simulink model "soc_pmsm_dualcpu_foc"  (R2023b)
settings: Solver=VariableStepAuto  StartTime=0.0  StopTime=.6  RelTol=1e-3  EnableMultiTasking=on
InitFcn:
  | soc_mcb_pmsm_foc_sensorless_f28379d_data;
model workspace (MAT data in the model file):
  mwTaskManagerKernelLatency = 0
values from neighbouring files (symbols this model uses):
  inverter = mcb_SetInverterParameters('BoostXL-DRV8305')    [soc_mcb_pmsm_foc_sensorless_f28379d_data.m]
  pmsm = mcb_SetPMSMMotorParameters('custom')    [soc_mcb_pmsm_foc_sensorless_f28379d_data.m]
  PU_System = mcb_SetPUSystem(pmsm,inverter)    [soc_mcb_pmsm_foc_sensorless_f28379d_data.m]
  PWM_frequency = 20e3    (= 20000)    [soc_mcb_pmsm_foc_sensorless_f28379d_data.m]
  Ts_motor = T_pwm/2    (= 2.5e-05)    [soc_mcb_pmsm_foc_sensorless_f28379d_data.m]
undefined symbols (not defined in the file or in its folder): D1, D2, Down, m, n, P, Up
libraries: fl_lib x50, nesl_utility x15, ee_lib x11, peripheralslib x5, procinterlib x2, proctasklib x2, mcbplantlib x1, mcbpositiondecoderlib x1, autolibpmsmexterior x1
(part 1 of 2)
settings Model: ExtModeTrigDuration=8  Creator=The MathWorks, Inc.  LastModifiedBy=The MathWorks, Inc.
settings SolverCC: AlgebraicLoopSolver=TrustRegion  PositivePriorityOrder=on  MaxZcPerStep=1
settings DataIOCC: SaveOutput=off  DSMLogging=off
settings OptimizationCC: DefaultUnderspecifiedDataType=single  EnhancedBackFolding=on  PassReuseOutputArgsAs=Individual arguments  MaxStackSize=1024  OptimizeBlockOrder=speed  DifferentSizesBufferReuse=on  OptimizationCustomize=off  DenormalBehavior=FlushToZero  EfficientTunableParamExpr=on
settings DebuggingCC: ParameterPrecisionLossMsg=none  ParameterTunabilityLossMsg=error  UnconnectedInputMsg=warning  UnconnectedOutputMsg=warning  UnconnectedLineMsg=warning
settings HardwareCC: ProdBitPerChar=16  ProdBitPerInt=16  ProdBitPerPointer=32  ProdBitPerSizeT=32  ProdBitPerPtrDiffT=32  ProdLargestAtomicInteger=Integer  ProdLargestAtomicFloat=None  ProdWordSize=16  ProdLongLongMode=on  ProdHWDeviceType=Texas Instruments->C2000  HardwareBoardFeatureSet=SoCBlockset
settings ModelReferenceCC: EnableRefExpFcnMdlSchedulingChecks=on
settings SFSimCC: MATLABDynamicMemAlloc=off
settings RTWCC: Description=Embedded Coder  SystemTargetFile=ert.tlc  HardwareBoard=TI Delfino F28379D LaunchPad  TLCOptions="-aInlineSetEventsForThisBaseRateFcn=TLC_FALSE -aSuppressMultiTaskScheduler=TLC_FALSE   -aRateBasedStepFcn=1"  TemplateMakefile=ert_default_tmf  Toolchain=Texas Instruments Code Composer Studio (C2000)  DLArmComputeVersion=19.05
settings CodeAppCC: ForceParamTrailComments=on  IgnoreCustomStorageClasses=off  OperatorAnnotations=on  SimulinkDataObjDesc=on  SFDataObjDesc=on  InsertBlockDesc=on
settings ERTTargetCC: CodeReplacementLibrary=TI C28x  ExtModeStaticAllocSize=10000

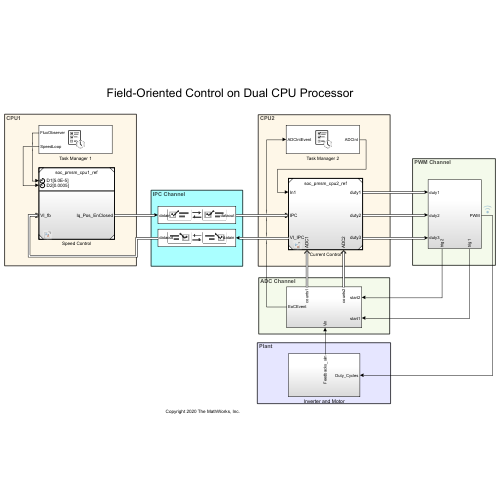
[thumbnail: Simulink's stored preview of the top-level diagram]
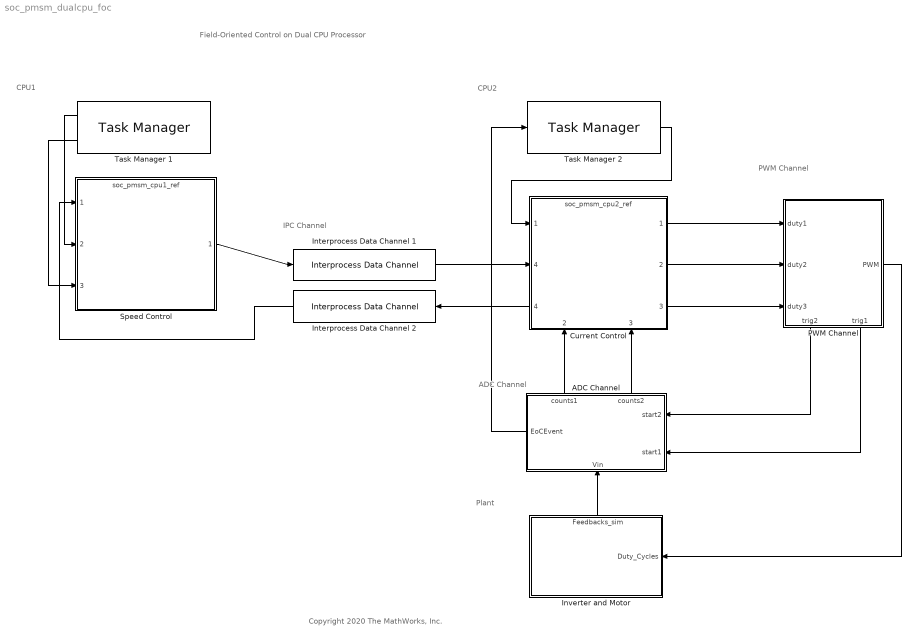
== system soc_pmsm_dualcpu_foc ==
  note: Field-Oriented Control on Dual CPU Processor
  note: CPU1
  note: PWM Channel
  note: IPC Channel
  note: CPU2
  note: Plant
  note: ADC Channel
  note: Copyright 2020 The MathWorks, Inc.
  ADC Channel : Subsystem
      settings: PortSchema="{\"entries\":[{\"content\":{\"sides\":[{\"content\":{\"connectorIds\":[\"In1\"]},\"type\":\"ConnectorPlacement.EquallySpacedRectSide\",\"uuid\":\"667350c5-41cd-4cba-abc8-8d5d0ac94845\"},{\"content\":{\"connectorIds\":[\"Out1\",\"Out2\"],\"side\":\"RIGHT\"},\"type\":\"ConnectorPlacement.EquallySpacedRectSide\",\"uuid\":\"5a172c81-9350-4ccc-b7f4-df82d7eca1de\"},{\"content\":{\"connectorIds\":[\"Out3\"],\"side\":\"TOP\"},\"type\":\"ConnectorPlacement.EquallySpacedRectSide\",\"uuid\":\"3830ed3a-e235-4bdf-8511-f25666678fd6\"},{\"content\":{\"connectorIds\":[\"In2\",\"In3\"],\"side\":\"BOTTOM\"},\"type\":\"ConnectorPlacement.EquallySpacedRectSide\",\"uuid\":\"15f45d0c-0c23-40c1-aa04-14d3d7fcf92d\"},{\"content\":{\"connectorIds\":[],\"side\":\"HIDDEN\"},\"type\":\"ConnectorPlacement.EquallySpacedRectSide\",\"uuid\":\"ee7e5474-69fd-4152-9972-ad3b7eda0b9e\"}]},\"type\":\"ConnectorPlacement.EquallySpacedConnector\",\"uuid\":\"8c4cca9e-82dc-4501-bb7e-3f52a3bf47b4\"}],\"packageUris\":[\"http://schema.mathworks.com/mf0/Connector/R2020b\"],\"version\":\"1.0\"}"
  Current Control : ModelReference  InputPortMessageModes=n,m,m,m  OutputPortMessageModes=m,m,m,m  ModelNameDialog=soc_pmsm_cpu2_ref.slx  SimulationMode=Normal  CachedPortDiscreteRates=[0.2]  ModelReferenceVersion=8.0
      settings: PortSchema="{\"entries\":[{\"content\":{\"sides\":[{\"content\":{\"connectorIds\":[\"In1\",\"In4\",\"Out4\"]},\"type\":\"ConnectorPlacement.EquallySpacedRectSide\",\"uuid\":\"9fd2c24c-ae51-46e5-a431-71bc240ed721\"},{\"content\":{\"connectorIds\":[\"Out1\",\"Out2\",\"Out3\"],\"side\":\"RIGHT\"},\"type\":\"ConnectorPlacement.EquallySpacedRectSide\",\"uuid\":\"f0a0e173-5aee-453c-b1bd-b370cde086ab\"},{\"content\":{\"connectorIds\":[],\"side\":\"TOP\"},\"type\":\"ConnectorPlacement.EquallySpacedRectSide\",\"uuid\":\"79c8d290-c938-4b10-a214-67592e778693\"},{\"content\":{\"connectorIds\":[\"In2\",\"In3\"],\"side\":\"BOTTOM\"},\"type\":\"ConnectorPlacement.EquallySpacedRectSide\",\"uuid\":\"f9ab5770-0d25-45e9-9b4a-55a67569c63a\"},{\"content\":{\"connectorIds\":[],\"side\":\"HIDDEN\"},\"type\":\"ConnectorPlacement.EquallySpacedRectSide\",\"uuid\":\"b923878a-78df-441a-99e2-7ad72d4d69ab\"}]},\"type\":\"ConnectorPlacement.EquallySpacedConnector\",\"uuid\":\"a5006b0b-636b-4340-a85c-125b87b251fa\"}],\"packageUris\":[\"http://schema.mathworks.com/mf0/Connector/R2020b\"],\"version\":\"1.0\"}"
  Interprocess Data Channel 1 : procinterlib/Interprocess Data Channel  NumBuffers=1  PropagationDelay=0  ShowEventPort=off  ShowNumUsedBuffers=off  ShowBufferOverwritten=off
  Interprocess Data Channel 2 : procinterlib/Interprocess Data Channel  NumBuffers=1  PropagationDelay=0  ShowEventPort=off  ShowNumUsedBuffers=off  ShowBufferOverwritten=off
  Inverter and Motor : Subsystem
      settings: PortSchema="{\"entries\":[{\"content\":{\"sides\":[{\"content\":{\"connectorIds\":[\"In1\"]},\"type\":\"ConnectorPlacement.EquallySpacedRectSide\",\"uuid\":\"958970e8-f51f-4be6-a255-39048d8abc04\"},{\"content\":{\"connectorIds\":[],\"side\":\"RIGHT\"},\"type\":\"ConnectorPlacement.EquallySpacedRectSide\",\"uuid\":\"a7d67471-63de-4fa9-8929-71ac779bb3a0\"},{\"content\":{\"connectorIds\":[\"Out1\"],\"side\":\"TOP\"},\"type\":\"ConnectorPlacement.EquallySpacedRectSide\",\"uuid\":\"f6853a86-6c38-405e-966d-f0bd0978db63\"},{\"content\":{\"connectorIds\":[],\"side\":\"HIDDEN\"},\"type\":\"ConnectorPlacement.EquallySpacedRectSide\",\"uuid\":\"0017b626-46a9-47f1-bc71-1e5fb05a995f\"}]},\"type\":\"ConnectorPlacement.EquallySpacedConnector\",\"uuid\":\"d320a7cc-19d6-4ac2-b759-0c9b58a9d13f\"}],\"packageUris\":[\"http://schema.mathworks.com/mf0/Connector/R2020b\"],\"version\":\"1.0\"}"
  PWM Channel : Subsystem
      settings: PortSchema="{\"entries\":[{\"content\":{\"sides\":[{\"content\":{\"connectorIds\":[\"In1\",\"In2\",\"In3\"]},\"type\":\"ConnectorPlacement.EquallySpacedRectSide\",\"uuid\":\"93269d63-2f51-4397-8262-c0fba5a35fbc\"},{\"content\":{\"connectorIds\":[\"Out1\"],\"side\":\"RIGHT\"},\"type\":\"ConnectorPlacement.EquallySpacedRectSide\",\"uuid\":\"01a9fb74-5fff-4873-a961-955e91d37141\"},{\"content\":{\"connectorIds\":[],\"side\":\"TOP\"},\"type\":\"ConnectorPlacement.EquallySpacedRectSide\",\"uuid\":\"96774146-0690-4e4a-a90b-a04dbe81855e\"},{\"content\":{\"connectorIds\":[\"Out2\",\"Out3\"],\"side\":\"BOTTOM\"},\"type\":\"ConnectorPlacement.EquallySpacedRectSide\",\"uuid\":\"cc316efe-bea7-4750-8d36-9fcd57c23279\"},{\"content\":{\"connectorIds\":[],\"side\":\"HIDDEN\"},\"type\":\"ConnectorPlacement.EquallySpacedRectSide\",\"uuid\":\"75c797b2-ef98-4bb8-8ad0-83cc5de0a8e5\"}]},\"type\":\"ConnectorPlacement.EquallySpacedConnector\",\"uuid\":\"6875c10b-95f0-453b-a724-f824d2af4c4b\"}],\"packageUris\":[\"http://schema.mathworks.com/mf0/Connector/R2020b\"],\"version\":\"1.0\"}"
  Speed Control : ModelReference  InputPortMessageModes=m,n,n  OutputPortMessageModes=m  ModelNameDialog=soc_pmsm_cpu1_ref.slx  SimulationMode=Normal  ScheduleRates=on  CachedPortDiscreteRates=[5.0E-5;0.0005]  ModelEventPortInfo=P:D1[5.0E-5][0][0],P:D2[0.0005][0][0]  ModelReferenceVersion=8.0
  Task Manager 1 : proctasklib/Task Manager  AllTaskData="[{\"taskName\":\"FluxObserver\",\"taskType\":\"Timer-driven\",\"taskEvent\":\"SpeedEvent\",\"taskPeriod\":\"Ts\",\"taskPriority\":\"50\",\"coreSelection\":\"Specified core\",\"coreNum\":\"0\",\"dropOverranTasks\":false,\"playbackRecorded\":false,\"diagnosticsFile\":\"\",\"taskDurationSource\":\"Dialog\",\"taskDuration\":1E-6,\"taskDurationDeviation\":0,\"logExecutionData\":true,\"logDroppedTasks\":false,\"version\":\"2.6\",\"taskDurationData\":{\"percent\":\"100\",\"mean\":\"1e-06\",\"dev\":\"0\",\"min\":\"1e-06\",\"max\":\"1e-06\"},\"taskEventSource\":\"Internal\",\"taskEventSourceAssignmentType\":\"AutoAssigned\",\"taskEventSourceType\":\"Unspecified\",\"taskEventGroup\":\"Unspecified\",\"taskEventInterrupt\":\"Unspecified\",\"taskEventOrder\":1,\"taskDisablePremption\":false,\"taskClearInterruptFlagsAtEndOfEvent\":false},{\"taskName\":\"SpeedLoop\",\"taskType\":\"Timer-driven\",\"taskEvent\":\"newTask1Event\",\"taskPeriod\":\"Ts_speed\",\"taskPriority\":\"50\",\"coreSelection\":\"Specified core\",\"coreNum\":\"0\",\"dropOverranTasks\":false,\"playbackRecorded\":false,\"diagnosticsFile\":\"\",\"taskDurationSource\":\"Dialog\",\"taskDuration\":1E-6,\"taskDurationDeviation\":0,\"logExecutionData\":true,\"logDroppedTasks\":false,\"version\":\"2.6\",\"taskDurationData\":{\"percent\":\"100\",\"mean\":\"1e-06\",\"dev\":\"0\",\"min\":\"1e-06\",\"max\":\"1e-06\"},\"taskEventSource\":\"Internal\",\"taskEventSourceAssignmentType\":\"AutoAssigned\",\"taskEventSourceType\":\"Unspecified\",\"taskEventGroup\":\"Unspecified\",\"taskEventInterrupt\":\"Unspecified\",\"taskEventOrder\":1,\"taskDisablePremption\":false,\"taskClearInterruptFlagsAtEndOfEvent\":false}]"  EnableTaskSimulation=off  StreamToSDI=on  WriteToFile=off  OverwriteFile=off  SupportEventPorts=on  UseScheduleEditor=off  CustomizationInfo=''
  Task Manager 2 : proctasklib/Task Manager  AllTaskData="{\"taskName\":\"ADCInt\",\"taskType\":\"Event-driven\",\"taskEvent\":\"ADCIntEvent\",\"taskPeriod\":\"0.1\",\"taskPriority\":\"50\",\"coreSelection\":\"Specified core\",\"coreNum\":\"0\",\"dropOverranTasks\":false,\"playbackRecorded\":false,\"diagnosticsFile\":\"\",\"taskDurationSource\":\"Dialog\",\"taskDuration\":1E-6,\"taskDurationDeviation\":0,\"logExecutionData\":true,\"logDroppedTasks\":false,\"version\":\"2.6\",\"taskDurationData\":{\"percent\":\"100\",\"mean\":\"1e-06\",\"dev\":\"0\",\"min\":\"1e-06\",\"max\":\"1e-06\"},\"taskEventSource\":\"EOC event\",\"taskEventSourceAssignmentType\":\"ManuallyAssigned\",\"taskEventSourceType\":\"Unspecified\",\"taskEventGroup\":\"ADC - Analog to Digital Converter\",\"taskEventInterrupt\":\"ADCB1_INT\",\"taskEventOrder\":1,\"taskDisablePremption\":false,\"taskClearInterruptFlagsAtEndOfEvent\":false}"  EnableTaskSimulation=off  StreamToSDI=on  WriteToFile=off  OverwriteFile=off  SupportEventPorts=on  UseScheduleEditor=off  CustomizationInfo=''
  wires:
  Speed Control/1 -> Interprocess Data Channel 1/1
  Interprocess Data Channel 2/1 -> Speed Control/1
  PWM Channel/1(PWM) -> Inverter and Motor/1(Duty_Cycles)
  ADC Channel/3(EoCEvent) -> Task Manager 2/1
  Task Manager 2/1 -> Current Control/1
  PWM Channel/2(trig2) -> ADC Channel/3(start2)
  PWM Channel/3(trig1) -> ADC Channel/2(start1)
  Interprocess Data Channel 1/1 -> Current Control/4
  Inverter and Motor/1(Feedbacks_sim) -> ADC Channel/1(Vin)
  ADC Channel/1(counts1) -> Current Control/2
  ADC Channel/2(counts2) -> Current Control/3
  Current Control/4 -> Interprocess Data Channel 2/1
  Current Control/1 -> PWM Channel/1(duty1)
  Current Control/2 -> PWM Channel/2(duty2)
  Current Control/3 -> PWM Channel/3(duty3)
  Task Manager 1/1 -> Speed Control/2
  Task Manager 1/2 -> Speed Control/3

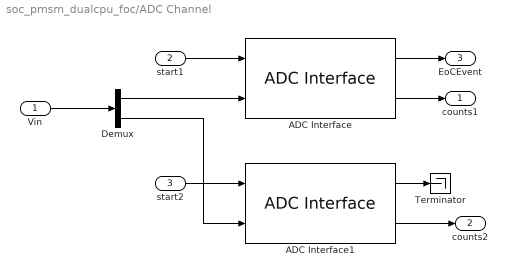
== system soc_pmsm_dualcpu_foc/ADC Channel ==
  Vin : Inport
  start1 : Inport  Port=2
  start2 : Inport  Port=3
  ADC Interface : peripheralslib/ADC Interface  ADCResolution=12  HighVref=3  AcqTime=320e-9  ConvTime=240e-9  TimeConstant=40e-9  SoftTrig=off  SampleTime=1e-3  NumCh=1  ConvType=Sequential  EnInterrupt=on  IntCondition=Acquisition + Conversion time  EnWatchdog=off  LowThreshold=.1  HighThreshold=2.9  IntLatency=0
  ADC Interface1 : peripheralslib/ADC Interface  ADCResolution=12  HighVref=3  AcqTime=320e-9  ConvTime=240e-9  TimeConstant=40e-9  SoftTrig=off  SampleTime=1e-3  NumCh=1  ConvType=Sequential  EnInterrupt=on  IntCondition=Acquisition + Conversion time  EnWatchdog=off  LowThreshold=.1  HighThreshold=2.9  IntLatency=0
  Demux : Demux  Outputs=2
  Terminator : Terminator
  counts1 : Outport
  counts2 : Outport  Port=2
  EoCEvent : Outport  Port=3
  wires:
  start1/1 -> ADC Interface/1
  start2/1 -> ADC Interface1/1
  Demux/2 -> ADC Interface1/2
  Vin/1 -> Demux/1
  Demux/1 -> ADC Interface/2
  ADC Interface1/2 -> counts2/1
  ADC Interface1/1 -> Terminator/1
  ADC Interface/2 -> counts1/1
  ADC Interface/1 -> EoCEvent/1

== system soc_pmsm_dualcpu_foc/Inverter and Motor ==
  Duty_Cycles : Inport
  Average or Switching : Subsystem  Variant=on  VariantControlMode=label  LabelModeActiveChoice=AverageInverter
  Feedbacks_sim : Outport  VectorParamsAs1DForOutWhenUnconnected=off
  wires:
  Average or Switching/1(Feedbacks_sim) -> Feedbacks_sim/1
  Duty_Cycles/1 -> Average or Switching/1(Duty_Cycles)

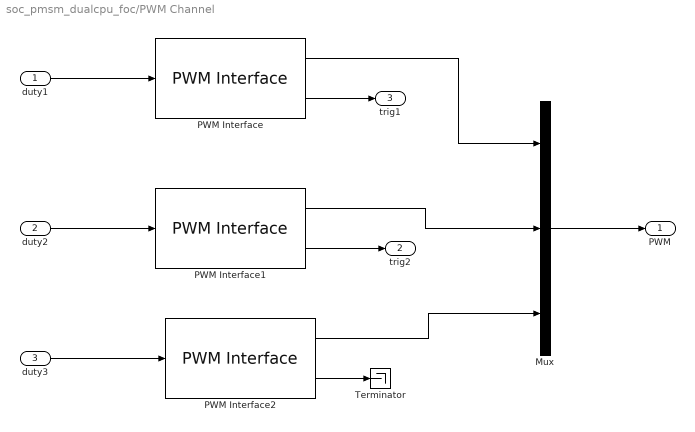
== system soc_pmsm_dualcpu_foc/PWM Channel ==
  duty1 : Inport
  duty2 : Inport  Port=2
  duty3 : Inport  Port=3
  Mux : Mux  Inputs=3
  PWM Interface : peripheralslib/PWM Interface  Period=1/PWM_frequency  OutSigMode=Average  CounterMode=Up-Down  GenCompPWM=off  DeadTimeTopPWM=100e-9  DeadTimeBottomPWM=100e-9  EventCondition2=End of PWM period  DataType=single  PWMAtStartPeriod=High  PWMAtMidPeriod=NoChange  PWMAtCMP1=Low  PWMAtCMP1UpCnt=Low  PWMAtCMP1DwnCnt=High  PWMAtCMP2=NoChange  PWMAtCMP2UpCnt=NoChange  PWMAtCMP2DwnCnt=NoChange  OutCountDir=off  PhaseOffset=0  EventType=ADC start  EventCondition1=Mid of PWM period  NumADCSOCToWait=1st event  NumADCSOCReplica=1  InterruptCond=End of PWM period  IntLatency=0  NumInterruptToWait=1st event
      settings: SamplingMode=End of PWM period
  PWM Interface1 : peripheralslib/PWM Interface  Period=1/PWM_frequency  OutSigMode=Average  CounterMode=Up-Down  GenCompPWM=off  DeadTimeTopPWM=100e-9  DeadTimeBottomPWM=100e-9  EventCondition2=End of PWM period  DataType=single  PWMAtStartPeriod=High  PWMAtMidPeriod=NoChange  PWMAtCMP1=Low  PWMAtCMP1UpCnt=Low  PWMAtCMP1DwnCnt=High  PWMAtCMP2=NoChange  PWMAtCMP2UpCnt=NoChange  PWMAtCMP2DwnCnt=NoChange  OutCountDir=off  PhaseOffset=0  EventType=ADC start  EventCondition1=Mid of PWM period  NumADCSOCToWait=1st event  NumADCSOCReplica=1  InterruptCond=End of PWM period  IntLatency=0  NumInterruptToWait=1st event
      settings: SamplingMode=End of PWM period
  PWM Interface2 : peripheralslib/PWM Interface  Period=1/PWM_frequency  OutSigMode=Average  CounterMode=Up-Down  GenCompPWM=off  DeadTimeTopPWM=100e-9  DeadTimeBottomPWM=100e-9  EventCondition2=End of PWM period  DataType=single  PWMAtStartPeriod=High  PWMAtMidPeriod=NoChange  PWMAtCMP1=Low  PWMAtCMP1UpCnt=Low  PWMAtCMP1DwnCnt=High  PWMAtCMP2=NoChange  PWMAtCMP2UpCnt=NoChange  PWMAtCMP2DwnCnt=NoChange  OutCountDir=off  PhaseOffset=0  EventType=ADC start  EventCondition1=Mid of PWM period  NumADCSOCToWait=1st event  NumADCSOCReplica=1  InterruptCond=End of PWM period  IntLatency=0  NumInterruptToWait=1st event
      settings: SamplingMode=End of PWM period
  Terminator : Terminator
  PWM : Outport
  trig2 : Outport  Port=2
  trig1 : Outport  Port=3
  wires:
  PWM Interface/2 -> trig1/1
  PWM Interface1/2 -> trig2/1
  PWM Interface2/2 -> Terminator/1
  Mux/1 -> PWM/1
  PWM Interface/1 -> Mux/1
  PWM Interface1/1 -> Mux/2
  PWM Interface2/1 -> Mux/3
  duty1/1 -> PWM Interface/1
  duty2/1 -> PWM Interface1/1
  duty3/1 -> PWM Interface2/1

== system soc_pmsm_dualcpu_foc/Inverter and Motor/Average or Switching ==
  note: 1) Add Subsystem or Model blocks as valid variant choices.
      | 2) You cannot connect blocks at this level. At simulation, connectivity is automatically
      | determined, based on the active variant and port name matching.
  Duty_Cycles : Inport
  Average : Subsystem  VariantControl=AverageInverter
  Switching : Subsystem  VariantControl=SwitchingInverter
  Feedbacks_sim : Outport  VectorParamsAs1DForOutWhenUnconnected=off

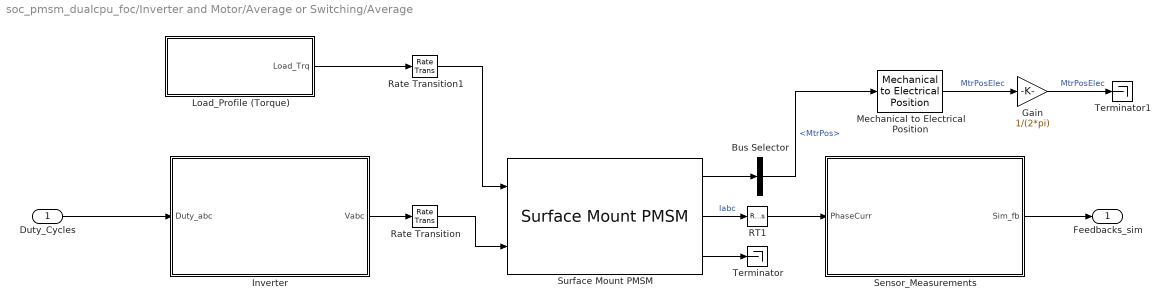
== system soc_pmsm_dualcpu_foc/Inverter and Motor/Average or Switching/Average ==
  Duty_Cycles : Inport
  Bus Selector : BusSelector  OutputSignals=MtrPos
  Gain : Gain  Gain=1/(2*pi)  OutDataTypeStr=Inherit: Same as input
  Inverter : Subsystem
  Load_Profile (Torque) : Subsystem
  Mechanical to Electrical Position : mcbpositiondecoderlib/Mechanical to Electrical Position  PolePairsInputType=Specify via dialog  NrPP=pmsm.p  selectedRange=Radians  MechOfstInputType=Specify via dialog  mechOffsetIn=0  maxAngleIn=2*pi  InputDataType=single  VariantSelect=floating-point
  RT1 : RateTransition  Deterministic=off  OutPortSampleTime=Ts_simulink
  Rate Transition : RateTransition  Deterministic=off  OutPortSampleTime=Ts_motor
  Rate Transition1 : RateTransition  Deterministic=off  OutPortSampleTime=Ts_motor
  Sensor_Measurements : Subsystem
  Surface Mount PMSM : autolibpmsmexterior/Surface Mount PMSM  port_config=Torque  sim_type=Discrete  Ts=Ts_motor  FilePath=surfacepmsm_motordata.m  P=pmsm.p  Rs=pmsm.Rs + inverter.R_board  Ldq_=pmsm.Ld  KConstText=Permanent flux linkage constant (lambda_pm):  lambda_pm=pmsm.FluxPM  Ke=159.9771  Kt=1.323  mechanical=[pmsm.J, pmsm.B, 0]  idq0=[0 0]  theta_init=0  omega_init=0  KConst=pmsm.FluxPM  lambda_pm_calc=pmsm.FluxPM  RefBlkName='autolibpmsmexterior/Surface Mount PMSM'  aMode=5  Ldq="[0.0002      0.0002]"
  Terminator : Terminator
  Terminator1 : Terminator
  Feedbacks_sim : Outport  VectorParamsAs1DForOutWhenUnconnected=off
  wires:
  Rate Transition/1 -> Surface Mount PMSM/2
  Gain/1 -> Terminator1/1  "MtrPosElec"
  Inverter/1(Vabc) -> Rate Transition/1
  Load_Profile (Torque)/1(Load_Trq) -> Rate Transition1/1
  RT1/1 -> Sensor_Measurements/1(PhaseCurr)
  Surface Mount PMSM/1 -> Bus Selector/1
  Bus Selector/1 -> Mechanical to Electrical Position/1  "<MtrPos>"
  Duty_Cycles/1 -> Inverter/1(Duty_abc)
  Surface Mount PMSM/2 -> RT1/1  "Iabc"
  Mechanical to Electrical Position/1 -> Gain/1  "MtrPosElec"
  Sensor_Measurements/1(Sim_fb) -> Feedbacks_sim/1
  Rate Transition1/1 -> Surface Mount PMSM/1
  Surface Mount PMSM/3 -> Terminator/1

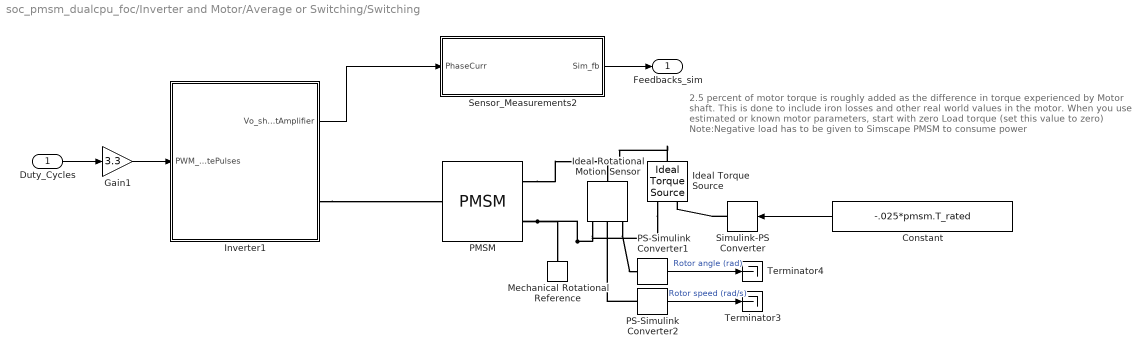
== system soc_pmsm_dualcpu_foc/Inverter and Motor/Average or Switching/Switching ==
  note: 2.5 percent of motor torque is roughly added as the difference in torque experienced by Motor shaft. This is done to include iron losses and other real world values in the motor.
      |
      | When you use estimated or known motor parameters, start with zero Load torque (set this value to zero)
      |
      | Note:Negative load has to be given to  Simscape PMSM to consume power
  Duty_Cycles : Inport
  Constant : Constant  Value=-.025*pmsm.T_rated  OutDataTypeStr=double
  Gain1 : Gain  Gain=3.3
  Ideal Rotational Motion Sensor : fl_lib/Mechanical/Mechanical Sensors/Ideal Rotational Motion Sensor  reference=foundation.enum.MeasurementReference.difference  acceleration_port=false  velocity_port=true  position_port=true  wrap_angle=simscape.enum.onoff.off  offset=0 deg
  Ideal Torque Source : fl_lib/Mechanical/Mechanical Sources/Ideal Torque Source
  Inverter1 : Subsystem
  Mechanical Rotational Reference : fl_lib/Mechanical/Rotational Elements/Mechanical Rotational Reference
  PMSM : ee_lib/Electromechanical/Permanent Magnet/PMSM  port_option=ee.enum.threePhasePort.composite  winding_type=ee.enum.statorconnection.wye  machine_param=ee.enum.pmsm.parameterization.constant  nPolePairs=pmsm.p  pmflux_param=ee.enum.pmflux.fluxlinkage  pm_flux_linkage=pmsm.FluxPM Wb  torque_constant=0.18 N*m/A  back_emf_constant=0.18 V/(rad/s)  stator_param=ee.enum.statorparam.LdLqL0  Ld=pmsm.Ld H  Lq=pmsm.Ld H  idVec=[-200, 0, 200] A  iqVec=[-200, 0, 200] A  LdMatrix=0.0002 * ones(3, 3) H  LqMatrix=0.0002 * ones(3, 3) H  PmMatrix=0.1 * ones(3, 3) Wb  ktMatrix=0.18 * ones(3, 3) N*m/A  keMatrix=0.18 * ones(3, 3) V/(rad/s)  L0=0 H  Ls=0.0002 H  Lm=-0.00002 H  Ms=0.00002 H  Rs=pmsm.Rs + inverter.R_board Ohm  zero_sequence=ee.enum.park.zerosequence.exclude  axes_param=ee.enum.rotorangle.daxis  loss_param=ee.enum.ironloss.none  losses_oc=[0, 0, 0] W  losses_sc=[0, 0, 0] W  f_losses=60 Hz  Isc_losses=95 A  J=pmsm.J kg*m^2  lam=pmsm.B N*m/(rad/s)  i_d_specify=off  i_d_priority=None  i_d=0 A  i_d_nominal_specify=off  i_d_nominal_unit=A  i_d_nominal_value=1  i_q_specify=off  i_q_priority=None  i_q=0 A  i_q_nominal_specify=off  i_q_nominal_unit=A  i_q_nominal_value=1  torque_specify=off  torque_priority=None  torque=0 N*m  torque_nominal_specify=off  torque_nominal_unit=N*m  torque_nominal_value=1  angular_velocity_specify=off  angular_velocity_priority=High  angular_velocity=0 rpm  angular_velocity_nominal_specify=off  angular_velocity_nominal_unit=rpm  angular_velocity_nominal_value=1  angular_position_specify=off  angular_position_priority=High  angular_position=0 deg  angular_position_nominal_specify=off  angular_position_nominal_unit=deg  angular_position_nominal_value=1  alpha=3.93e-3 1/K  alpha_flux=-0.001 1/K  Tmeas=298.15 K  stator_thermal_mass=100 J/K  rotor_thermal_mass=200 J/K  Rm_percent_rotor=90  Rd_percent_rotor=30  temperatureA_specify=off  temperatureA_priority=High  temperatureA=25 degC  temperatureA_nominal_specify=off  temperatureA_nominal_unit=degC  temperatureA_nominal_value=1  temperatureB_specify=off  temperatureB_priority=High  temperatureB=25 degC  temperatureB_nominal_specify=off  temperatureB_nominal_unit=degC  temperatureB_nominal_value=1  temperatureC_specify=off  temperatureC_priority=High  temperatureC=25 degC  temperatureC_nominal_specify=off  temperatureC_nominal_unit=degC  temperatureC_nominal_value=1  temperatureR_specify=off  temperatureR_priority=High  temperatureR=25 degC  temperatureR_nominal_specify=off  temperatureR_nominal_unit=degC  temperatureR_nominal_value=1
      settings: InternalSimscapePortConfiguration="{\"Bottom\":[],\"Left\":[{\"id\":\"N\",\"label\":\"~\",\"type\":\"foundation.electrical.three_phase\"}],\"Right\":[{\"id\":\"R\",\"label\":\"R\",\"type\":\"foundation.mechanical.rotational.rotational\"},{\"id\":\"C\",\"label\":\"C\",\"type\":\"foundation.mechanical.rotational.rotational\"}],\"Top\":[]}"
  PS-Simulink Converter1 : nesl_utility/PS-Simulink Converter  PhysicalDomain=network_engine_domain  SubClassName=ps_output  LeftPortType=input  RightPortType=output  PseudoPeriodic=off  Frequencies=[]  VectorFormat=1-D array  Unit=rad  AffineConversion=off
  PS-Simulink Converter2 : nesl_utility/PS-Simulink Converter  PhysicalDomain=network_engine_domain  SubClassName=ps_output  LeftPortType=input  RightPortType=output  PseudoPeriodic=off  Frequencies=[]  VectorFormat=1-D array  Unit=rad/s  AffineConversion=off
  Sensor_Measurements2 : Subsystem
  Simulink-PS Converter : nesl_utility/Simulink-PS Converter  PhysicalDomain=network_engine_domain  SubClassName=ps_input  LeftPortType=input  RightPortType=output  PseudoPeriodic=off  Frequencies=[]  NoiseDistribution=none  NoiseParameters=[]  Unit=1  AffineConversion=off  FilteringAndDerivatives=provide  SimscapeFilterOrder=1  InputFilterTimeConstant=0.001  UdotUserProvided=0
  Terminator3 : Terminator
  Terminator4 : Terminator
  Feedbacks_sim : Outport  VectorParamsAs1DForOutWhenUnconnected=off
  wires:
  Inverter1/1(Vo_shuntAmplifier) -> Sensor_Measurements2/1(PhaseCurr)
  Gain1/1 -> Inverter1/1(PWM_GatePulses)
  PS-Simulink Converter2/1 -> Terminator3/1  "Rotor speed (rad/s)"
  PS-Simulink Converter1/1 -> Terminator4/1  "Rotor angle (rad)"
  Duty_Cycles/1 -> Gain1/1
  Sensor_Measurements2/1(Sim_fb) -> Feedbacks_sim/1
  Constant/1 -> Simulink-PS Converter/1
  connections:
  PMSM/RConn1 -- Ideal Rotational Motion Sensor/LConn1 -- Ideal Torque Source/LConn1
  PMSM/RConn2 -- Mechanical Rotational Reference/LConn1 -- Ideal Rotational Motion Sensor/RConn1 -- Ideal Torque Source/RConn2
  PS-Simulink Converter2/LConn1 -- Ideal Rotational Motion Sensor/RConn2
  Inverter1/RConn1 -- PMSM/LConn1
  Ideal Rotational Motion Sensor/RConn3 -- PS-Simulink Converter1/LConn1
  Simulink-PS Converter/RConn1 -- Ideal Torque Source/RConn1

== system soc_pmsm_dualcpu_foc/Inverter and Motor/Average or Switching/Average/Inverter ==
  Duty_abc : Inport
  Average-Value Inverter : mcbplantlib/Average-Value Inverter
  Constant2 : Constant  Value=inverter.V_dc  OutDataTypeStr=single  SampleTime=-1
  Data Type Conversion1 : DataTypeConversion  OutDataTypeStr=single  RndMeth=Simplest  SaturateOnIntegerOverflow=off
  Rate Transition3 : RateTransition  Deterministic=off  OutPortSampleTime=Ts_inverter
  Vabc : Outport  VectorParamsAs1DForOutWhenUnconnected=off
  wires:
  Data Type Conversion1/1 -> Rate Transition3/1
  Duty_abc/1 -> Data Type Conversion1/1
  Rate Transition3/1 -> Average-Value Inverter/1
  Constant2/1 -> Average-Value Inverter/2
  Average-Value Inverter/1 -> Vabc/1

== system soc_pmsm_dualcpu_foc/Inverter and Motor/Average or Switching/Average/Load_Profile (Torque) ==
  note: 2.5 percent of motor torque is roughly added as the difference in torque experienced by Motor shaft. This is done to include iron losses and other real world values in the motor.
      |
      | When you use estimated or known motor parameters, start with zero Load torque (set this value to zero)
  Constant : Constant  Value=.025*pmsm.T_rated  OutDataTypeStr=single
  Load_Trq : Outport  VectorParamsAs1DForOutWhenUnconnected=off
  wires:
  Constant/1 -> Load_Trq/1

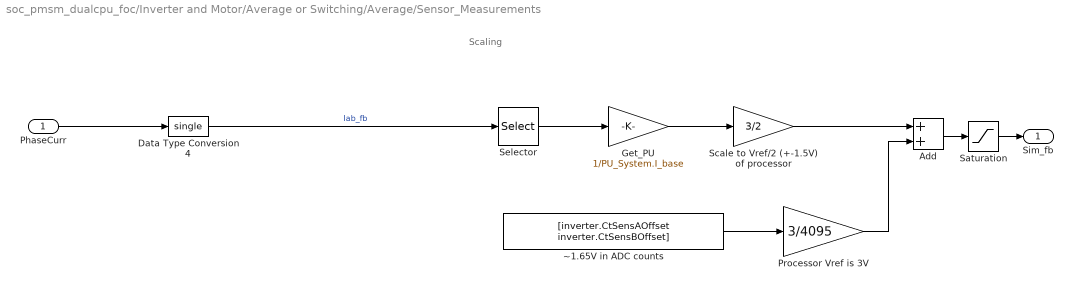
== system soc_pmsm_dualcpu_foc/Inverter and Motor/Average or Switching/Average/Sensor_Measurements ==
  note: Scaling
  PhaseCurr : Inport
  Add : Sum
  Data Type Conversion4 : DataTypeConversion  OutDataTypeStr=single  RndMeth=Simplest  SaturateOnIntegerOverflow=off
  Get_PU : Gain  Gain=1/PU_System.I_base  RndMeth=Simplest
  Processor Vref is 3V : Gain  Gain=3/4095  OutDataTypeStr=single
  Saturation : Saturate  UpperLimit=3.3  LowerLimit=0
  Scale to Vref/2 (+-1.5V) of processor : Gain  Gain=3/2  RndMeth=Simplest  OutDataTypeStr=Inherit: Same as input
  Selector : Selector  InputPortWidth=3  IndexOptions=Index vector (dialog)  Indices=[1 2]  OutputSizes=1
  ~1.65V in ADC counts : Constant  Value=[inverter.CtSensAOffset inverter.CtSensBOffset]  OutDataTypeStr=uint16  SampleTime=-1
  Sim_fb : Outport  VectorParamsAs1DForOutWhenUnconnected=off
  wires:
  Add/1 -> Saturation/1
  ~1.65V in ADC counts/1 -> Processor Vref is 3V/1
  Data Type Conversion4/1 -> Selector/1  "Iab_fb"
  Selector/1 -> Get_PU/1
  PhaseCurr/1 -> Data Type Conversion4/1
  Get_PU/1 -> Scale to Vref/2 (+-1.5V) of processor/1
  Processor Vref is 3V/1 -> Add/2
  Saturation/1 -> Sim_fb/1
  Scale to Vref/2 (+-1.5V) of processor/1 -> Add/1

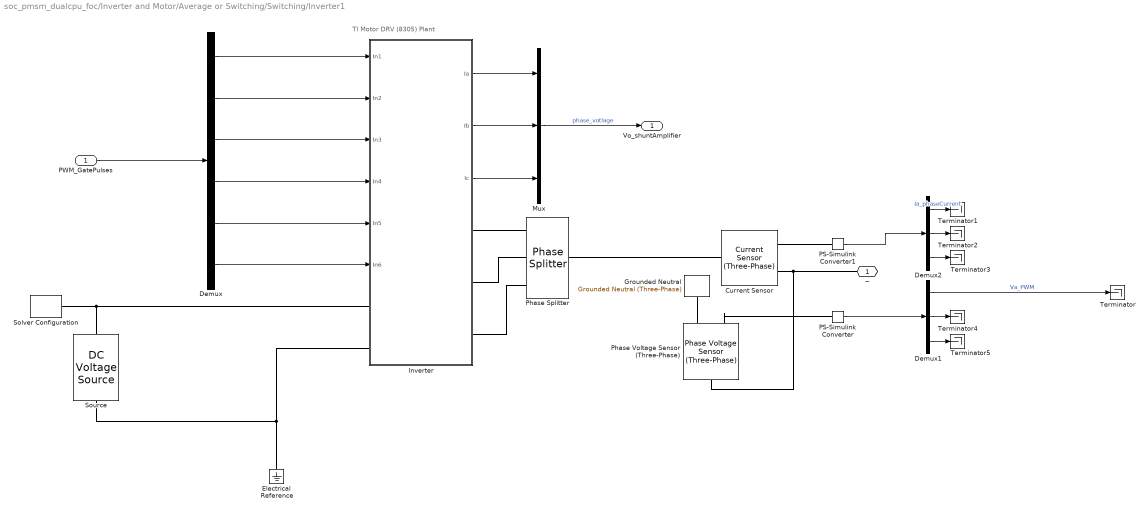
== system soc_pmsm_dualcpu_foc/Inverter and Motor/Average or Switching/Switching/Inverter1 ==
  note: TI Motor DRV (8305) Plant
  PWM_GatePulses : Inport
  Current Sensor : ee_lib/Sensors & Transducers/Current Sensor (Three-Phase)
  Demux : Demux  Outputs=6
  Demux1 : Demux  Outputs=3
  Demux2 : Demux  Outputs=3
  Electrical Reference : fl_lib/Electrical/Electrical Elements/Electrical Reference
  Grounded Neutral : ee_lib/Connectors & References/Grounded Neutral (Three-Phase)
  Inverter : Subsystem
  Mux : Mux  Inputs=3
  PS-Simulink Converter : nesl_utility/PS-Simulink Converter  PhysicalDomain=network_engine_domain  SubClassName=ps_output  LeftPortType=input  RightPortType=output  PseudoPeriodic=off  Frequencies=[]  VectorFormat=1-D array  Unit=1  AffineConversion=off
  PS-Simulink Converter1 : nesl_utility/PS-Simulink Converter  PhysicalDomain=network_engine_domain  SubClassName=ps_output  LeftPortType=input  RightPortType=output  PseudoPeriodic=off  Frequencies=[]  VectorFormat=1-D array  Unit=1  AffineConversion=off
  Phase Splitter : ee_lib/Connectors & References/Phase Splitter
  Phase Voltage Sensor (Three-Phase) : ee_lib/Sensors & Transducers/Phase Voltage Sensor (Three-Phase)
  Solver Configuration : nesl_utility/Solver Configuration  PhysicalDomain=network_engine_domain  SubClassName=solver  LeftPortType=input  RightPortType=generic  Tones=[]  Harmonics=[]  SimulateNoise=off  Profile=off  UseLocalSampling=off  EnableSwitchedLinearOptims=on  FrequencyDomain=off  UseCCode=off  RelTol=0.001  AbsTol=1e-06  MinStep=1e-09  ToWorkspace=off  RevertToSquareIcSolve=off  NumHomotopyIterations=100  PhasorMode=off  PhasorModeNumHarmonics=1  ConsistencySolver=NEWTON_FTOL  IndexReductionMethod=DerivativeReplacement  DoDC=off  ResidualTolerance=1e-09  ConsistencyTolSource=GLOBAL  ConsistencyAbsTol=0.001  ConsistencyRelTol=0.001  ConsistencyTolFactor=0.001  UseLocalSolver=off  LocalSolverChoice=NE_BACKWARD_EULER_ADVANCER  ResolveIndetEquations=on  FunctionEvalNumThread=1  LocalSolverSampleTime=.5e-6  DoFixedCost=off  MaxNonlinIter=3  MaxModeIter=2  ComputeImpulses=off  ImpulseIterations=1  LinearAlgebra=auto  LinearAlgebraNumThread=0  EquationFormulation=NE_TIME_EF  DelaysMemoryBudget=1024  AutomaticFiltering=on  FilteringTimeConstant=0.001  PartitionStorageMethod=AS_NEEDED  PartitionMemoryBudget=1024  PartitionMethod=ROBUST  MultibodyUseLocalSolver=off  MultibodyLocalSolverChoice=ODE1  MultibodyLocalSolverSampleTime=0.001
  Source : fl_lib/Electrical/Electrical Sources/DC Voltage Source  v0=inverter.V_dc V
  Terminator{,1..5} (6 alike) : Terminator
  ~ : PMIOPort  Side=Right
  Vo_shuntAmplifier : Outport  VectorParamsAs1DForOutWhenUnconnected=off
  wires:
  PWM_GatePulses/1 -> Demux/1
  Mux/1 -> Vo_shuntAmplifier/1  "phase_votlage"
  PS-Simulink Converter/1 -> Demux1/1
  PS-Simulink Converter1/1 -> Demux2/1
  Demux2/1 -> Terminator1/1  "Ia_phaseCurrent"
  Inverter/3(Ic) -> Mux/3
  Inverter/1(Ia) -> Mux/1
  Inverter/2(Ib) -> Mux/2
  Demux2/2 -> Terminator2/1
  Demux2/3 -> Terminator3/1
  Demux1/2 -> Terminator4/1
  Demux1/3 -> Terminator5/1
  Demux1/1 -> Terminator/1  "Va_PWM"
  Demux/1 -> Inverter/1(In1)
  Demux/2 -> Inverter/2(In2)
  Demux/3 -> Inverter/3(In3)
  Demux/4 -> Inverter/4(In4)
  Demux/5 -> Inverter/5(In5)
  Demux/6 -> Inverter/6(In6)
  connections:
  Current Sensor/LConn1 -- Phase Splitter/LConn1
  Grounded Neutral/LConn1 -- Phase Voltage Sensor (Three-Phase)/RConn2
  Phase Voltage Sensor (Three-Phase)/RConn1 -- PS-Simulink Converter/LConn1
  Current Sensor/RConn1 -- PS-Simulink Converter1/LConn1
  Source/LConn1 -- Solver Configuration/RConn1 -- Inverter/LConn1
  Electrical Reference/LConn1 -- Inverter/LConn2 -- Source/RConn1
  ~/RConn1 -- Phase Voltage Sensor (Three-Phase)/LConn1 -- Current Sensor/RConn2
  Inverter/RConn3 -- Phase Splitter/RConn3
  Inverter/RConn2 -- Phase Splitter/RConn2
  Inverter/RConn1 -- Phase Splitter/RConn1

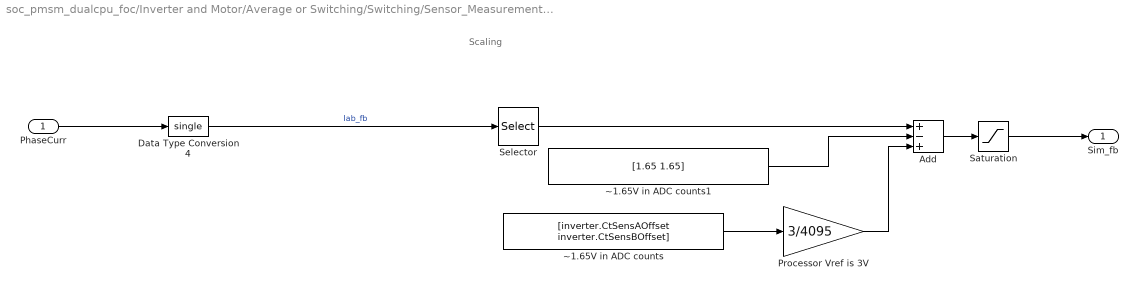
== system soc_pmsm_dualcpu_foc/Inverter and Motor/Average or Switching/Switching/Sensor_Measurements2 ==
  note: Scaling
  PhaseCurr : Inport
  Add : Sum  Inputs=+-+
  Data Type Conversion4 : DataTypeConversion  OutDataTypeStr=single  RndMeth=Simplest  SaturateOnIntegerOverflow=off
  Processor Vref is 3V : Gain  Gain=3/4095  OutDataTypeStr=single
  Saturation : Saturate  UpperLimit=3  LowerLimit=0
  Selector : Selector  InputPortWidth=3  IndexOptions=Index vector (dialog)  Indices=[1 2]  OutputSizes=1
  ~1.65V in ADC counts : Constant  Value=[inverter.CtSensAOffset inverter.CtSensBOffset]  OutDataTypeStr=uint16  SampleTime=-1
  ~1.65V in ADC counts1 : Constant  Value=[1.65 1.65]  OutDataTypeStr=single  SampleTime=-1
  Sim_fb : Outport  VectorParamsAs1DForOutWhenUnconnected=off
  wires:
  Add/1 -> Saturation/1
  ~1.65V in ADC counts/1 -> Processor Vref is 3V/1
  Data Type Conversion4/1 -> Selector/1  "Iab_fb"
  PhaseCurr/1 -> Data Type Conversion4/1
  Saturation/1 -> Sim_fb/1
  Selector/1 -> Add/1
  Processor Vref is 3V/1 -> Add/3
  ~1.65V in ADC counts1/1 -> Add/2

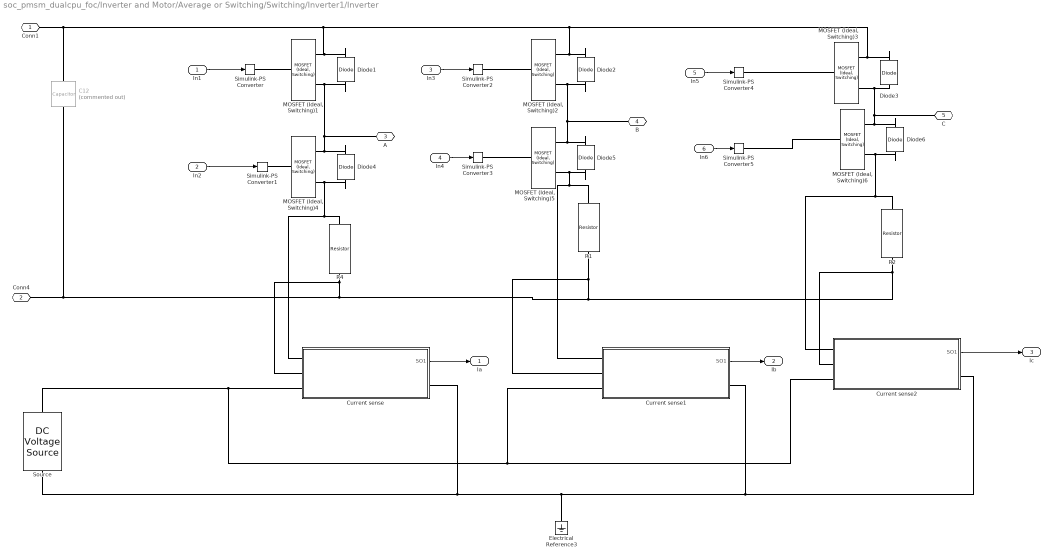
== system soc_pmsm_dualcpu_foc/Inverter and Motor/Average or Switching/Switching/Inverter1/Inverter ==
  In1 : Inport
  In2 : Inport  Port=2
  In3 : Inport  Port=3
  In4 : Inport  Port=4
  In5 : Inport  Port=5
  In6 : Inport  Port=6
  C12 : fl_lib/Electrical/Electrical Elements/Capacitor  Commented=on  c=5000 pF  r=1e-6 Ohm  g=0 1/Ohm  i_specify=off  i_priority=None  i=0 A  i_nominal_specify=off  i_nominal_unit=A  i_nominal_value=1  v_specify=off  v_priority=None  v=0 V  v_nominal_specify=off  v_nominal_unit=V  v_nominal_value=1  vc_specify=off  vc_priority=High  vc=0 V  vc_nominal_specify=off  vc_nominal_unit=V  vc_nominal_value=1
  Current sense : Subsystem
  Current sense1 : Subsystem
  Current sense2 : Subsystem
  Diode{1..6} (6 alike) : fl_lib/Electrical/Electrical Elements/Diode  Vf=.7 V  Ron=1e-6 Ohm  Goff=1e-8 1/Ohm  i_specify=off  i_priority=None  i=0 A  i_nominal_specify=off  i_nominal_unit=A  i_nominal_value=1  v_specify=off  v_priority=None  v=0 V  v_nominal_specify=off  v_nominal_unit=V  v_nominal_value=1
  Electrical Reference3 : fl_lib/Electrical/Electrical Elements/Electrical Reference
  MOSFET (Ideal, Switching){1..6} (6 alike) : ee_lib/Semiconductors & Converters/MOSFET (Ideal, Switching)  port_option=ee.enum.controlport.ps  Rds=2.6e-3 Ohm  Goff=1e-6 1/Ohm  Vth=2 V  diode_param=1  diode_Vf=0.8 V  diode_Ron=0.001 Ohm  diode_Goff=1e-5 1/Ohm  diode_C=50e-9 F  diode_iRM=-235 A  diode_iF=300 A  diode_idot=-50 A/us  diode_trr_param=1  diode_trr_factor=3  diode_trr=15 us  diode_Qrr=1500 s*uA  ids_specify=off  ids_priority=None  ids=0 A  ids_nominal_specify=off  ids_nominal_unit=A  ids_nominal_value=1  vds_specify=off  vds_priority=None  vds=0 V  vds_nominal_specify=off  vds_nominal_unit=V  vds_nominal_value=1  vgs_specify=off  vgs_priority=None  vgs=0 V  vgs_nominal_specify=off  vgs_nominal_unit=V  vgs_nominal_value=1  thermal_loss_option=ee.enum.converters.thermalLossOption.constantvalues  Von_data=[0, 1.8, 3.2, 6, 10, 16; 0, 2, 5.5, 9.5, 15, 25] V  Tj=[298.15, 448.15] K  Iout_data=[0, 20, 40, 60, 80, 100] A  Eon_data=[0, 55.04, 124.57, 235.53, 362.12; 0, 71.25, 161.25, 304.88, 468.75] * 1e-6 J  Eoff_data=[0, 18, 30, 56.1, 76.5; 0, 22.5, 37.5, 70.13, 95.63] * 1e-6 J  Eon_data_3D=[zeros(2, 5, 3)] J  Eoff_data_3D=[zeros(2, 5, 3)] J  Tj_loss=[298.15, 448.15] K  Iout_data_loss=[0, 10, 20, 30, 40] A  tabulateWithVds=false  Vds_loss=[0, 150, 300] V  Eon_scalar=22.86e-3 J  Eoff_scalar=17.14e-3 J  Voff=300 V  Iout_scalar=600 A  useCurrentFromPreviousCycle=false  useVoltageFromPreviousCycle=false  diodeModelType=ee.enum.converters.diodeModelType.pwl  diodeTableType=ee.enum.diode.tableType.IfMat  diode_IfMat=[.07, .12, .19, 1.75, 4.24, 7.32, 11.2; .16, .3, .72, 2.14, 4.02, 6.35, 9.12] A  diode_VfMat=[.9, 1.15, 1.25, 1.5, 1.75, 2.17, 2.6, 2.85; .58, .68, .75, 1.1, 1.38, 1.77, 2.27, 2.7] V  diode_TjVec=[25, 125] degC  diode_VfVec=[.5, .7, .9, 1.3, 1.7, 2.1, 2.5] V  diode_IfVec=[.1, .2, .5, 1, 2, 4, 7, 10] A  diode_Vr=-600 V  diode_Ls=150 nH  diode_Erec=0.03 J  diode_rec_loss_model=ee.enum.diode.reverseRecoveryModel.fixed  diode_ErecVal=0 J  diode_scaleWithIandV=true  diode_ErecMat=zeros(2, 3) J  diode_TjrecVec=[298.15, 398.15] K  diode_IfrecVec=[.1, 1, 10] A  diode_IrecVal=10 A  diode_VrecVal=10 V  diode_tFilter=1 / 1000 / 100 s  thermal_network_parameterization=ee.enum.thermalNetworkTopology.external  Rth=[.03, .2] K/W  Rth_Cauer=[.03, .1, .2] K/W  Rth_Foster=[.03, .2] K/W  thermal_mass_parameterization=ee.enum.thermalNetwork.timeconstant  thermal_mass=[3, 25] J/K  thermal_mass_Cauer=[3, 10, 25] J/K  thermal_mass_Foster=[33, 50] J/K  thermal_time_constant=[.1, 5] s  thermal_time_constant_Cauer=[.1, 1, 5] s  thermal_time_constant_Foster=[1, 10] s  thermal_mass_initial_temperatures=[25, 25] degC  thermal_mass_initial_temperatures_Cauer=[25, 25, 25] degC  junction_thermal_mass=0.1 J/K  Tvec_initial_Foster=[25, 25, 25, 25] degC  no_thermal_network=0  junction_temperature_specify=off  junction_temperature_priority=None  junction_temperature=25 degC  junction_temperature_nominal_specify=off  junction_temperature_nominal_unit=degC  junction_temperature_nominal_value=1  Qj_specify=off  Qj_priority=None  Qj=0 W  Qj_nominal_specify=off  Qj_nominal_unit=W  Qj_nominal_value=1  accumulatedSwitchingLosses_specify=off  accumulatedSwitchingLosses_priority=None  accumulatedSwitchingLosses=0 J
  R1 : fl_lib/Electrical/Electrical Elements/Resistor  R=.007 Ohm  i_specify=off  i_priority=None  i=0 A  i_nominal_specify=off  i_nominal_unit=A  i_nominal_value=1  v_specify=off  v_priority=None  v=0 V  v_nominal_specify=off  v_nominal_unit=V  v_nominal_value=1
  R2 : fl_lib/Electrical/Electrical Elements/Resistor  R=.007 Ohm  i_specify=off  i_priority=None  i=0 A  i_nominal_specify=off  i_nominal_unit=A  i_nominal_value=1  v_specify=off  v_priority=None  v=0 V  v_nominal_specify=off  v_nominal_unit=V  v_nominal_value=1
  R4 : fl_lib/Electrical/Electrical Elements/Resistor  R=.007 Ohm  i_specify=off  i_priority=None  i=0 A  i_nominal_specify=off  i_nominal_unit=A  i_nominal_value=1  v_specify=off  v_priority=None  v=0 V  v_nominal_specify=off  v_nominal_unit=V  v_nominal_value=1
  Simulink-PS Converter{,1..5} (6 alike) : nesl_utility/Simulink-PS Converter  PhysicalDomain=network_engine_domain  SubClassName=ps_input  LeftPortType=input  RightPortType=output  PseudoPeriodic=off  Frequencies=[]  NoiseDistribution=none  NoiseParameters=[]  Unit=1  AffineConversion=off  FilteringAndDerivatives=provide  SimscapeFilterOrder=1  InputFilterTimeConstant=0.001  UdotUserProvided=0
  Source : fl_lib/Electrical/Electrical Sources/DC Voltage Source  v0=3.3 V
  Conn1 : PMIOPort  Side=Left
  Conn4 : PMIOPort  Port=2  Side=Left
  A : PMIOPort  Port=3  Side=Right
  B : PMIOPort  Port=4  Side=Right
  C : PMIOPort  Port=5  Side=Right
  Ia : Outport  VectorParamsAs1DForOutWhenUnconnected=off
  Ib : Outport  Port=2  VectorParamsAs1DForOutWhenUnconnected=off
  Ic : Outport  Port=3  VectorParamsAs1DForOutWhenUnconnected=off
  wires:
  In5/1 -> Simulink-PS Converter4/1
  In4/1 -> Simulink-PS Converter3/1
  In3/1 -> Simulink-PS Converter2/1
  In2/1 -> Simulink-PS Converter1/1
  Current sense1/1(SO1) -> Ib/1
  Current sense/1(SO1) -> Ia/1
  Current sense2/1(SO1) -> Ic/1
  In6/1 -> Simulink-PS Converter5/1
  In1/1 -> Simulink-PS Converter/1
  connections:
  Diode4/LConn1 -- Current sense/LConn1 -- R4/LConn1 -- "MOSFET (Ideal, Switching)4"/RConn2
  Conn4/RConn1 -- R1/RConn1 -- Current sense1/LConn2 -- Current sense2/LConn2 -- R2/RConn1 -- R4/RConn1 -- Current sense/LConn2 -- C12/RConn1
  Diode5/LConn1 -- R1/LConn1 -- Current sense1/LConn1 -- "MOSFET (Ideal, Switching)5"/RConn2
  Diode6/LConn1 -- R2/LConn1 -- Current sense2/LConn1 -- "MOSFET (Ideal, Switching)6"/RConn2
  Current sense1/LConn3 -- Current sense2/LConn3 -- Current sense/LConn3 -- Source/LConn1
  Current sense1/RConn1 -- Current sense2/RConn1 -- Electrical Reference3/LConn1 -- Source/RConn1 -- Current sense/RConn1
  Diode2/RConn1 -- "MOSFET (Ideal, Switching)1"/RConn1 -- Diode1/RConn1 -- C12/LConn1 -- Conn1/RConn1 -- "MOSFET (Ideal, Switching)3"/RConn1 -- Diode3/RConn1 -- "MOSFET (Ideal, Switching)2"/RConn1
  Diode4/RConn1 -- "MOSFET (Ideal, Switching)1"/RConn2 -- Diode1/LConn1 -- A/RConn1 -- "MOSFET (Ideal, Switching)4"/RConn1
  Diode5/RConn1 -- B/RConn1 -- "MOSFET (Ideal, Switching)2"/RConn2 -- Diode2/LConn1 -- "MOSFET (Ideal, Switching)5"/RConn1
  Simulink-PS Converter/RConn1 -- "MOSFET (Ideal, Switching)1"/LConn1
  Simulink-PS Converter1/RConn1 -- "MOSFET (Ideal, Switching)4"/LConn1
  "MOSFET (Ideal, Switching)5"/LConn1 -- Simulink-PS Converter3/RConn1
  Diode6/RConn1 -- C/RConn1 -- Diode3/LConn1 -- "MOSFET (Ideal, Switching)3"/RConn2 -- "MOSFET (Ideal, Switching)6"/RConn1
  Simulink-PS Converter4/RConn1 -- "MOSFET (Ideal, Switching)3"/LConn1
  Simulink-PS Converter5/RConn1 -- "MOSFET (Ideal, Switching)6"/LConn1
  Simulink-PS Converter2/RConn1 -- "MOSFET (Ideal, Switching)2"/LConn1

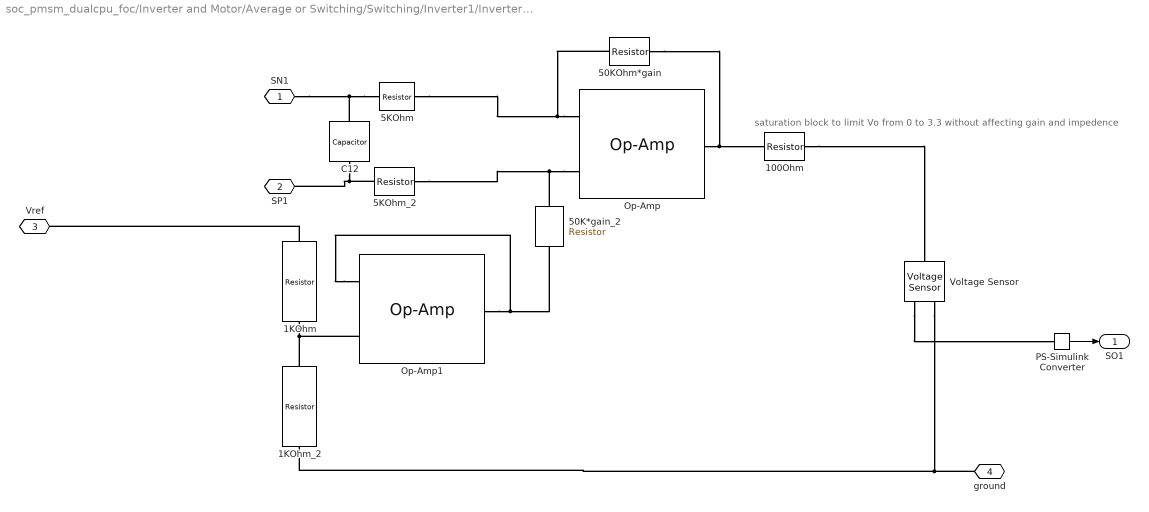
== system soc_pmsm_dualcpu_foc/Inverter and Motor/Average or Switching/Switching/Inverter1/Inverter/Current sense ==
  note: saturation block to limit Vo from 0 to 3.3 without affecting gain and impedence
  100Ohm : fl_lib/Electrical/Electrical Elements/Resistor  R=100 Ohm  i_specify=off  i_priority=None  i=0 A  i_nominal_specify=off  i_nominal_unit=A  i_nominal_value=1  v_specify=off  v_priority=None  v=0 V  v_nominal_specify=off  v_nominal_unit=V  v_nominal_value=1
  1KOhm : fl_lib/Electrical/Electrical Elements/Resistor  R=1 kOhm  i_specify=off  i_priority=None  i=0 A  i_nominal_specify=off  i_nominal_unit=A  i_nominal_value=1  v_specify=off  v_priority=None  v=0 V  v_nominal_specify=off  v_nominal_unit=V  v_nominal_value=1
  1KOhm_2 : fl_lib/Electrical/Electrical Elements/Resistor  R=1 kOhm  i_specify=off  i_priority=None  i=0 A  i_nominal_specify=off  i_nominal_unit=A  i_nominal_value=1  v_specify=off  v_priority=None  v=0 V  v_nominal_specify=off  v_nominal_unit=V  v_nominal_value=1
  50K*gain_2 : fl_lib/Electrical/Electrical Elements/Resistor  R=50*inverter.ADCGain kOhm  i_specify=off  i_priority=None  i=0 A  i_nominal_specify=off  i_nominal_unit=A  i_nominal_value=1  v_specify=off  v_priority=None  v=0 V  v_nominal_specify=off  v_nominal_unit=V  v_nominal_value=1
  50KOhm*gain : fl_lib/Electrical/Electrical Elements/Resistor  R=50*inverter.ADCGain kOhm  i_specify=off  i_priority=None  i=0 A  i_nominal_specify=off  i_nominal_unit=A  i_nominal_value=1  v_specify=off  v_priority=None  v=0 V  v_nominal_specify=off  v_nominal_unit=V  v_nominal_value=1
  5KOhm : fl_lib/Electrical/Electrical Elements/Resistor  R=5 kOhm  i_specify=off  i_priority=None  i=0 A  i_nominal_specify=off  i_nominal_unit=A  i_nominal_value=1  v_specify=off  v_priority=None  v=0 V  v_nominal_specify=off  v_nominal_unit=V  v_nominal_value=1
  5KOhm_2 : fl_lib/Electrical/Electrical Elements/Resistor  R=5 kOhm  i_specify=off  i_priority=None  i=0 A  i_nominal_specify=off  i_nominal_unit=A  i_nominal_value=1  v_specify=off  v_priority=None  v=0 V  v_nominal_specify=off  v_nominal_unit=V  v_nominal_value=1
  C12 : fl_lib/Electrical/Electrical Elements/Capacitor  c=1000 pF  r=1e-6 Ohm  g=0 1/Ohm  i_specify=off  i_priority=None  i=0 A  i_nominal_specify=off  i_nominal_unit=A  i_nominal_value=1  v_specify=off  v_priority=None  v=0 V  v_nominal_specify=off  v_nominal_unit=V  v_nominal_value=1  vc_specify=off  vc_priority=High  vc=0 V  vc_nominal_specify=off  vc_nominal_unit=V  vc_nominal_value=1
  Op-Amp : fl_lib/Electrical/Electrical Elements/Op-Amp  outI_specify=off  outI_priority=None  outI=0 A  outI_nominal_specify=off  outI_nominal_unit=A  outI_nominal_value=1
  Op-Amp1 : fl_lib/Electrical/Electrical Elements/Op-Amp  outI_specify=off  outI_priority=None  outI=0 A  outI_nominal_specify=off  outI_nominal_unit=A  outI_nominal_value=1
  PS-Simulink Converter : nesl_utility/PS-Simulink Converter  PhysicalDomain=network_engine_domain  SubClassName=ps_output  LeftPortType=input  RightPortType=output  PseudoPeriodic=off  Frequencies=[]  VectorFormat=1-D array  Unit=V  AffineConversion=off
  Voltage Sensor : fl_lib/Electrical/Electrical Sensors/Voltage Sensor
  SN1 : PMIOPort  Side=Left
  SP1 : PMIOPort  Port=2  Side=Left
  Vref : PMIOPort  Port=3  Side=Left
  ground : PMIOPort  Port=4  Side=Right
  SO1 : Outport  VectorParamsAs1DForOutWhenUnconnected=off
  wires:
  PS-Simulink Converter/1 -> SO1/1
  connections:
  100Ohm/RConn1 -- Voltage Sensor/LConn1
  Voltage Sensor/RConn1 -- PS-Simulink Converter/LConn1
  Voltage Sensor/RConn2 -- 1KOhm_2/RConn1 -- ground/RConn1
  5KOhm/LConn1 -- C12/LConn1 -- SN1/RConn1
  SP1/RConn1 -- C12/RConn1 -- 5KOhm_2/LConn1
  1KOhm/LConn1 -- Vref/RConn1
  Op-Amp/LConn1 -- 50K*gain_2/LConn1 -- 5KOhm_2/RConn1
  Op-Amp1/LConn2 -- 50K*gain_2/RConn1 -- Op-Amp1/RConn1
  Op-Amp/LConn2 -- 50KOhm*gain/LConn1 -- 5KOhm/RConn1
  50KOhm*gain/RConn1 -- 100Ohm/LConn1 -- Op-Amp/RConn1
  1KOhm/RConn1 -- Op-Amp1/LConn1 -- 1KOhm_2/LConn1

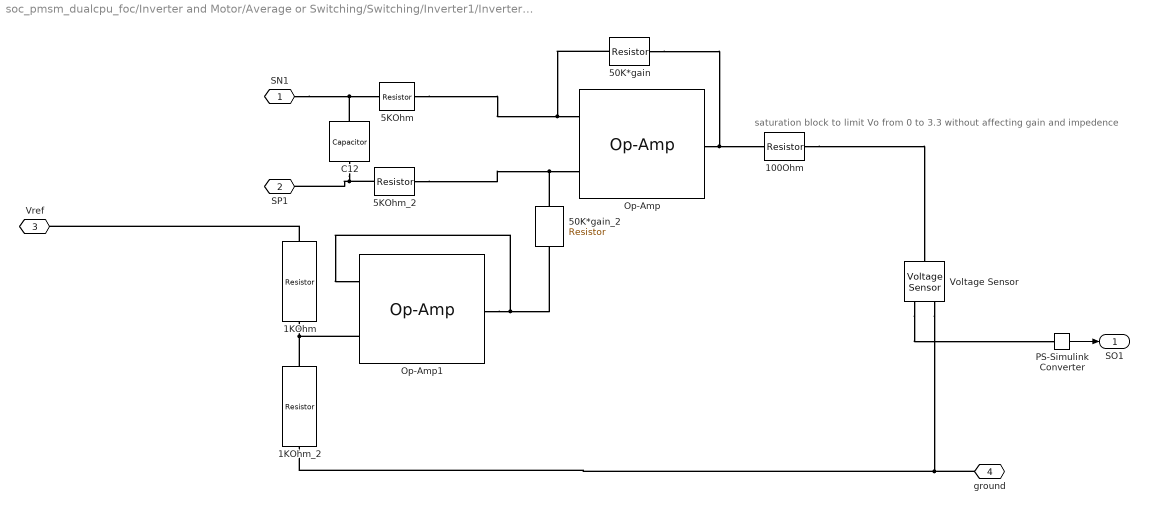
== system soc_pmsm_dualcpu_foc/Inverter and Motor/Average or Switching/Switching/Inverter1/Inverter/Current sense1 ==
  note: saturation block to limit Vo from 0 to 3.3 without affecting gain and impedence
  100Ohm : fl_lib/Electrical/Electrical Elements/Resistor  R=100 Ohm  i_specify=off  i_priority=None  i=0 A  i_nominal_specify=off  i_nominal_unit=A  i_nominal_value=1  v_specify=off  v_priority=None  v=0 V  v_nominal_specify=off  v_nominal_unit=V  v_nominal_value=1
  1KOhm : fl_lib/Electrical/Electrical Elements/Resistor  R=1 kOhm  i_specify=off  i_priority=None  i=0 A  i_nominal_specify=off  i_nominal_unit=A  i_nominal_value=1  v_specify=off  v_priority=None  v=0 V  v_nominal_specify=off  v_nominal_unit=V  v_nominal_value=1
  1KOhm_2 : fl_lib/Electrical/Electrical Elements/Resistor  R=1 kOhm  i_specify=off  i_priority=None  i=0 A  i_nominal_specify=off  i_nominal_unit=A  i_nominal_value=1  v_specify=off  v_priority=None  v=0 V  v_nominal_specify=off  v_nominal_unit=V  v_nominal_value=1
  50K*gain : fl_lib/Electrical/Electrical Elements/Resistor  R=50*inverter.ADCGain kOhm  i_specify=off  i_priority=None  i=0 A  i_nominal_specify=off  i_nominal_unit=A  i_nominal_value=1  v_specify=off  v_priority=None  v=0 V  v_nominal_specify=off  v_nominal_unit=V  v_nominal_value=1
  50K*gain_2 : fl_lib/Electrical/Electrical Elements/Resistor  R=50*inverter.ADCGain kOhm  i_specify=off  i_priority=None  i=0 A  i_nominal_specify=off  i_nominal_unit=A  i_nominal_value=1  v_specify=off  v_priority=None  v=0 V  v_nominal_specify=off  v_nominal_unit=V  v_nominal_value=1
  5KOhm : fl_lib/Electrical/Electrical Elements/Resistor  R=5 kOhm  i_specify=off  i_priority=None  i=0 A  i_nominal_specify=off  i_nominal_unit=A  i_nominal_value=1  v_specify=off  v_priority=None  v=0 V  v_nominal_specify=off  v_nominal_unit=V  v_nominal_value=1
  5KOhm_2 : fl_lib/Electrical/Electrical Elements/Resistor  R=5 kOhm  i_specify=off  i_priority=None  i=0 A  i_nominal_specify=off  i_nominal_unit=A  i_nominal_value=1  v_specify=off  v_priority=None  v=0 V  v_nominal_specify=off  v_nominal_unit=V  v_nominal_value=1
  C12 : fl_lib/Electrical/Electrical Elements/Capacitor  c=1000 pF  r=1e-6 Ohm  g=0 1/Ohm  i_specify=off  i_priority=None  i=0 A  i_nominal_specify=off  i_nominal_unit=A  i_nominal_value=1  v_specify=off  v_priority=None  v=0 V  v_nominal_specify=off  v_nominal_unit=V  v_nominal_value=1  vc_specify=off  vc_priority=High  vc=0 V  vc_nominal_specify=off  vc_nominal_unit=V  vc_nominal_value=1
  Op-Amp : fl_lib/Electrical/Electrical Elements/Op-Amp  outI_specify=off  outI_priority=None  outI=0 A  outI_nominal_specify=off  outI_nominal_unit=A  outI_nominal_value=1
  Op-Amp1 : fl_lib/Electrical/Electrical Elements/Op-Amp  outI_specify=off  outI_priority=None  outI=0 A  outI_nominal_specify=off  outI_nominal_unit=A  outI_nominal_value=1
  PS-Simulink Converter : nesl_utility/PS-Simulink Converter  PhysicalDomain=network_engine_domain  SubClassName=ps_output  LeftPortType=input  RightPortType=output  PseudoPeriodic=off  Frequencies=[]  VectorFormat=1-D array  Unit=V  AffineConversion=off
  Voltage Sensor : fl_lib/Electrical/Electrical Sensors/Voltage Sensor
  SN1 : PMIOPort  Side=Left
  SP1 : PMIOPort  Port=2  Side=Left
  Vref : PMIOPort  Port=3  Side=Left
  ground : PMIOPort  Port=4  Side=Right
  SO1 : Outport  VectorParamsAs1DForOutWhenUnconnected=off
  wires:
  PS-Simulink Converter/1 -> SO1/1
  connections:
  1KOhm_2/LConn1 -- Op-Amp1/LConn1 -- 1KOhm/RConn1
  Op-Amp/RConn1 -- 100Ohm/LConn1 -- 50K*gain/RConn1
  5KOhm/RConn1 -- 50K*gain/LConn1 -- Op-Amp/LConn2
  Op-Amp1/RConn1 -- 50K*gain_2/RConn1 -- Op-Amp1/LConn2
  5KOhm_2/RConn1 -- 50K*gain_2/LConn1 -- Op-Amp/LConn1
  1KOhm/LConn1 -- Vref/RConn1
  5KOhm_2/LConn1 -- C12/RConn1 -- SP1/RConn1
  SN1/RConn1 -- C12/LConn1 -- 5KOhm/LConn1
  ground/RConn1 -- Voltage Sensor/RConn2 -- 1KOhm_2/RConn1
  Voltage Sensor/RConn1 -- PS-Simulink Converter/LConn1
  100Ohm/RConn1 -- Voltage Sensor/LConn1
